simulink model "Seessin4_Scripting_Excersise3"  (R2014a)
settings: Solver=ode45  StartTime=0.0  StopTime=10.0  RelTol=1e-3
settings Model: Creator=Omar Emad  LastModifiedBy=Omar Emad

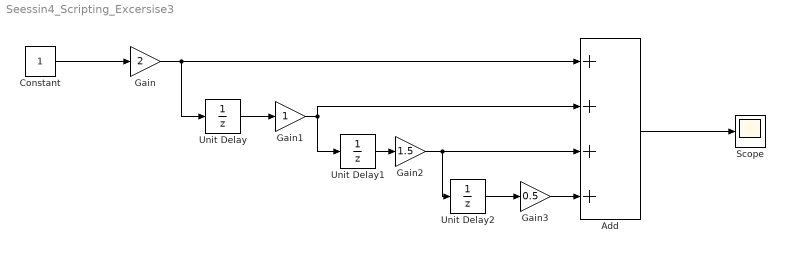
== system Seessin4_Scripting_Excersise3 ==
  Add : Sum  Inputs=++++
  Constant : Constant
  Gain : Gain  Gain=2  SampleTime=1
  Gain1 : Gain  SampleTime=2
  Gain2 : Gain  Gain=1.5  SampleTime=3
  Gain3 : Gain  Gain=0.5  SampleTime=4
  Scope : Scope
  Unit Delay : UnitDelay  SampleTime=-1
  Unit Delay1 : UnitDelay  SampleTime=-1
  Unit Delay2 : UnitDelay  SampleTime=-1
  wires:
  Constant/1 -> Gain/1
  Unit Delay/1 -> Gain1/1
  Unit Delay1/1 -> Gain2/1
  Unit Delay2/1 -> Gain3/1
  Add/1 -> Scope/1
  Gain/1 -> Add/1, Unit Delay/1
  Gain1/1 -> Add/2, Unit Delay1/1
  Gain2/1 -> Unit Delay2/1, Add/3
  Gain3/1 -> Add/4
